simulink model "LoFT_Example3"  (R2024b)
settings: Solver=ode4  StartTime=0.0  StopTime=300  FixedStep=simu.dt  RelTol=1e-3
undefined symbols (not defined in the file): body, circtime, Communication, D1, Delta, irkb, line, LoFT, p0, Pn, s, simu, trip_time, Turbwind, waves, wind
libraries: simulink x350, spsThreePhaseVIMeasurementLib x41, spsThreePhasePISectionLineLib x34, spsThreePhaseParallelRLCLoadLib x21, spsThreePhaseTransformerTwoWindingsLib x14, spsLoadFlowBusLib x10, spsThreePhaseDynamicLoadLib x9, spsSynchronousMachinepuStandardLib x7, spsExcitationSystemLib x7, spsSteamTurbineandGovernorLib x7, spsGenericPowerSystemStabilizerLib x7, spsMultiBandPowerSystemStabilizerLib x7
(part 10 of 49)

== system LoFT_Example3/FOWT System/Subsystem7/wave series 9 ==
  1-D Lookup Table : Lookup_n-D  NumberOfTableDimensions=1  BreakpointsForDimension1=LoFT.Hydro.waveforces.time + 10  Table=squeeze(LoFT.Hydro.waveforces.force(1,1,:))  InternalRulePriority=Speed  RndMeth=Simplest
  1-D Lookup Table1 : Lookup_n-D  NumberOfTableDimensions=1  BreakpointsForDimension1=LoFT.Hydro.waveforces.time + 10  Table=squeeze(LoFT.Hydro.waveforces.force(1,2,:))  InternalRulePriority=Speed  RndMeth=Simplest
  1-D Lookup Table2 : Lookup_n-D  NumberOfTableDimensions=1  BreakpointsForDimension1=LoFT.Hydro.waveforces.time + 10  Table=squeeze(LoFT.Hydro.waveforces.force(1,3,:))  InternalRulePriority=Speed  RndMeth=Simplest
  Clock1 : Clock
  Clock2 : Clock
  Clock3 : Clock
  Vector Concatenate1 : Concatenate  NumInputs=3
  Out1 : Outport
  wires:
  1-D Lookup Table2/1 -> Vector Concatenate1/3
  1-D Lookup Table1/1 -> Vector Concatenate1/2
  Clock1/1 -> 1-D Lookup Table/1
  Clock3/1 -> 1-D Lookup Table2/1
  1-D Lookup Table/1 -> Vector Concatenate1/1
  Clock2/1 -> 1-D Lookup Table1/1
  Vector Concatenate1/1 -> Out1/1

== system LoFT_Example3/FOWT System/Wind Conditions/wind series 1 ==
  Clock1 : Clock
  Lookup Table2 : Lookup_n-D  NumberOfTableDimensions=1  BreakpointsForDimension1=Turbwind.WF(1).Time  BreakpointsForDimension2=wind.yDiscr  BreakpointsForDimension3=wind.zDiscr  Table=Turbwind.WF(1).WindVelX  InternalRulePriority=Speed  RndMeth=Simplest
  Out1 : Outport
  wires:
  Lookup Table2/1 -> Out1/1
  Clock1/1 -> Lookup Table2/1

== system LoFT_Example3/FOWT System/Wind Conditions/wind series 10 ==
  Clock1 : Clock
  Lookup Table2 : Lookup_n-D  NumberOfTableDimensions=1  BreakpointsForDimension1=Turbwind.WF(1).Time  BreakpointsForDimension2=wind.yDiscr  BreakpointsForDimension3=wind.zDiscr  Table=Turbwind.WF(10).WindVelX  InternalRulePriority=Speed  RndMeth=Simplest
  Scope : Scope
  Out1 : Outport
  wires:
  Clock1/1 -> Lookup Table2/1
  Lookup Table2/1 -> Scope/1, Out1/1

== system LoFT_Example3/FOWT System/Wind Conditions/wind series 11 ==
  Clock1 : Clock
  Lookup Table2 : Lookup_n-D  NumberOfTableDimensions=1  BreakpointsForDimension1=Turbwind.WF(1).Time  BreakpointsForDimension2=wind.yDiscr  BreakpointsForDimension3=wind.zDiscr  Table=Turbwind.WF(11).WindVelX  InternalRulePriority=Speed  RndMeth=Simplest
  Out1 : Outport
  wires:
  Lookup Table2/1 -> Out1/1
  Clock1/1 -> Lookup Table2/1

== system LoFT_Example3/FOWT System/Wind Conditions/wind series 12 ==
  Clock1 : Clock
  Lookup Table2 : Lookup_n-D  NumberOfTableDimensions=1  BreakpointsForDimension1=Turbwind.WF(1).Time  BreakpointsForDimension2=wind.yDiscr  BreakpointsForDimension3=wind.zDiscr  Table=Turbwind.WF(12).WindVelX  InternalRulePriority=Speed  RndMeth=Simplest
  Out1 : Outport
  wires:
  Clock1/1 -> Lookup Table2/1
  Lookup Table2/1 -> Out1/1

== system LoFT_Example3/FOWT System/Wind Conditions/wind series 13 ==
  Clock1 : Clock
  Lookup Table2 : Lookup_n-D  NumberOfTableDimensions=1  BreakpointsForDimension1=Turbwind.WF(1).Time  BreakpointsForDimension2=wind.yDiscr  BreakpointsForDimension3=wind.zDiscr  Table=Turbwind.WF(13).WindVelX  InternalRulePriority=Speed  RndMeth=Simplest
  Out1 : Outport
  wires:
  Lookup Table2/1 -> Out1/1
  Clock1/1 -> Lookup Table2/1

== system LoFT_Example3/FOWT System/Wind Conditions/wind series 14 ==
  Clock1 : Clock
  Lookup Table2 : Lookup_n-D  NumberOfTableDimensions=1  BreakpointsForDimension1=Turbwind.WF(1).Time  BreakpointsForDimension2=wind.yDiscr  BreakpointsForDimension3=wind.zDiscr  Table=Turbwind.WF(14).WindVelX  InternalRulePriority=Speed  RndMeth=Simplest
  Out1 : Outport
  wires:
  Clock1/1 -> Lookup Table2/1
  Lookup Table2/1 -> Out1/1

== system LoFT_Example3/FOWT System/Wind Conditions/wind series 15 ==
  Clock1 : Clock
  Lookup Table2 : Lookup_n-D  NumberOfTableDimensions=1  BreakpointsForDimension1=Turbwind.WF(1).Time  BreakpointsForDimension2=wind.yDiscr  BreakpointsForDimension3=wind.zDiscr  Table=Turbwind.WF(15).WindVelX  InternalRulePriority=Speed  RndMeth=Simplest
  Out1 : Outport
  wires:
  Lookup Table2/1 -> Out1/1
  Clock1/1 -> Lookup Table2/1

== system LoFT_Example3/FOWT System/Wind Conditions/wind series 16 ==
  Clock1 : Clock
  Lookup Table2 : Lookup_n-D  NumberOfTableDimensions=1  BreakpointsForDimension1=Turbwind.WF(1).Time  BreakpointsForDimension2=wind.yDiscr  BreakpointsForDimension3=wind.zDiscr  Table=Turbwind.WF(16).WindVelX  InternalRulePriority=Speed  RndMeth=Simplest
  Out1 : Outport
  wires:
  Clock1/1 -> Lookup Table2/1
  Lookup Table2/1 -> Out1/1

== system LoFT_Example3/FOWT System/Wind Conditions/wind series 17 ==
  Clock1 : Clock
  Lookup Table2 : Lookup_n-D  NumberOfTableDimensions=1  BreakpointsForDimension1=Turbwind.WF(1).Time  BreakpointsForDimension2=wind.yDiscr  BreakpointsForDimension3=wind.zDiscr  Table=Turbwind.WF(17).WindVelX  InternalRulePriority=Speed  RndMeth=Simplest
  Out1 : Outport
  wires:
  Lookup Table2/1 -> Out1/1
  Clock1/1 -> Lookup Table2/1

== system LoFT_Example3/FOWT System/Wind Conditions/wind series 18 ==
  Clock1 : Clock
  Lookup Table2 : Lookup_n-D  NumberOfTableDimensions=1  BreakpointsForDimension1=Turbwind.WF(1).Time  BreakpointsForDimension2=wind.yDiscr  BreakpointsForDimension3=wind.zDiscr  Table=Turbwind.WF(18).WindVelX  InternalRulePriority=Speed  RndMeth=Simplest
  Out1 : Outport
  wires:
  Clock1/1 -> Lookup Table2/1
  Lookup Table2/1 -> Out1/1

== system LoFT_Example3/FOWT System/Wind Conditions/wind series 19 ==
  Clock1 : Clock
  Lookup Table2 : Lookup_n-D  NumberOfTableDimensions=1  BreakpointsForDimension1=Turbwind.WF(1).Time  BreakpointsForDimension2=wind.yDiscr  BreakpointsForDimension3=wind.zDiscr  Table=Turbwind.WF(19).WindVelX  InternalRulePriority=Speed  RndMeth=Simplest
  Out1 : Outport
  wires:
  Lookup Table2/1 -> Out1/1
  Clock1/1 -> Lookup Table2/1

== system LoFT_Example3/FOWT System/Wind Conditions/wind series 2 ==
  Clock1 : Clock
  Lookup Table2 : Lookup_n-D  NumberOfTableDimensions=1  BreakpointsForDimension1=Turbwind.WF(1).Time  BreakpointsForDimension2=wind.yDiscr  BreakpointsForDimension3=wind.zDiscr  Table=Turbwind.WF(2).WindVelX  InternalRulePriority=Speed  RndMeth=Simplest
  Out1 : Outport
  wires:
  Clock1/1 -> Lookup Table2/1
  Lookup Table2/1 -> Out1/1

== system LoFT_Example3/FOWT System/Wind Conditions/wind series 20 ==
  Clock1 : Clock
  Lookup Table2 : Lookup_n-D  NumberOfTableDimensions=1  BreakpointsForDimension1=Turbwind.WF(1).Time  BreakpointsForDimension2=wind.yDiscr  BreakpointsForDimension3=wind.zDiscr  Table=Turbwind.WF(20).WindVelX  InternalRulePriority=Speed  RndMeth=Simplest
  Scope : Scope
  Out1 : Outport
  wires:
  Lookup Table2/1 -> Out1/1, Scope/1
  Clock1/1 -> Lookup Table2/1

== system LoFT_Example3/FOWT System/Wind Conditions/wind series 21 ==
  Clock1 : Clock
  Lookup Table2 : Lookup_n-D  NumberOfTableDimensions=1  BreakpointsForDimension1=Turbwind.WF(1).Time  BreakpointsForDimension2=wind.yDiscr  BreakpointsForDimension3=wind.zDiscr  Table=Turbwind.WF(21).WindVelX  InternalRulePriority=Speed  RndMeth=Simplest
  Out1 : Outport
  wires:
  Lookup Table2/1 -> Out1/1
  Clock1/1 -> Lookup Table2/1

== system LoFT_Example3/FOWT System/Wind Conditions/wind series 22 ==
  Clock1 : Clock
  Lookup Table2 : Lookup_n-D  NumberOfTableDimensions=1  BreakpointsForDimension1=Turbwind.WF(1).Time  BreakpointsForDimension2=wind.yDiscr  BreakpointsForDimension3=wind.zDiscr  Table=Turbwind.WF(22).WindVelX  InternalRulePriority=Speed  RndMeth=Simplest
  Out1 : Outport
  wires:
  Clock1/1 -> Lookup Table2/1
  Lookup Table2/1 -> Out1/1

== system LoFT_Example3/FOWT System/Wind Conditions/wind series 23 ==
  Clock1 : Clock
  Lookup Table2 : Lookup_n-D  NumberOfTableDimensions=1  BreakpointsForDimension1=Turbwind.WF(1).Time  BreakpointsForDimension2=wind.yDiscr  BreakpointsForDimension3=wind.zDiscr  Table=Turbwind.WF(23).WindVelX  InternalRulePriority=Speed  RndMeth=Simplest
  Out1 : Outport
  wires:
  Lookup Table2/1 -> Out1/1
  Clock1/1 -> Lookup Table2/1

== system LoFT_Example3/FOWT System/Wind Conditions/wind series 24 ==
  Clock1 : Clock
  Lookup Table2 : Lookup_n-D  NumberOfTableDimensions=1  BreakpointsForDimension1=Turbwind.WF(1).Time  BreakpointsForDimension2=wind.yDiscr  BreakpointsForDimension3=wind.zDiscr  Table=Turbwind.WF(24).WindVelX  InternalRulePriority=Speed  RndMeth=Simplest
  Out1 : Outport
  wires:
  Clock1/1 -> Lookup Table2/1
  Lookup Table2/1 -> Out1/1

== system LoFT_Example3/FOWT System/Wind Conditions/wind series 25 ==
  Clock1 : Clock
  Lookup Table2 : Lookup_n-D  NumberOfTableDimensions=1  BreakpointsForDimension1=Turbwind.WF(1).Time  BreakpointsForDimension2=wind.yDiscr  BreakpointsForDimension3=wind.zDiscr  Table=Turbwind.WF(25).WindVelX  InternalRulePriority=Speed  RndMeth=Simplest
  Out1 : Outport
  wires:
  Lookup Table2/1 -> Out1/1
  Clock1/1 -> Lookup Table2/1

== system LoFT_Example3/FOWT System/Wind Conditions/wind series 26 ==
  Clock1 : Clock
  Lookup Table2 : Lookup_n-D  NumberOfTableDimensions=1  BreakpointsForDimension1=Turbwind.WF(1).Time  BreakpointsForDimension2=wind.yDiscr  BreakpointsForDimension3=wind.zDiscr  Table=Turbwind.WF(26).WindVelX  InternalRulePriority=Speed  RndMeth=Simplest
  Out1 : Outport
  wires:
  Clock1/1 -> Lookup Table2/1
  Lookup Table2/1 -> Out1/1

== system LoFT_Example3/FOWT System/Wind Conditions/wind series 27 ==
  Clock1 : Clock
  Lookup Table2 : Lookup_n-D  NumberOfTableDimensions=1  BreakpointsForDimension1=Turbwind.WF(1).Time  BreakpointsForDimension2=wind.yDiscr  BreakpointsForDimension3=wind.zDiscr  Table=Turbwind.WF(27).WindVelX  InternalRulePriority=Speed  RndMeth=Simplest
  Out1 : Outport
  wires:
  Lookup Table2/1 -> Out1/1
  Clock1/1 -> Lookup Table2/1

== system LoFT_Example3/FOWT System/Wind Conditions/wind series 28 ==
  Clock1 : Clock
  Lookup Table2 : Lookup_n-D  NumberOfTableDimensions=1  BreakpointsForDimension1=Turbwind.WF(1).Time  BreakpointsForDimension2=wind.yDiscr  BreakpointsForDimension3=wind.zDiscr  Table=Turbwind.WF(28).WindVelX  InternalRulePriority=Speed  RndMeth=Simplest
  Out1 : Outport
  wires:
  Clock1/1 -> Lookup Table2/1
  Lookup Table2/1 -> Out1/1

== system LoFT_Example3/FOWT System/Wind Conditions/wind series 29 ==
  Clock1 : Clock
  Lookup Table2 : Lookup_n-D  NumberOfTableDimensions=1  BreakpointsForDimension1=Turbwind.WF(1).Time  BreakpointsForDimension2=wind.yDiscr  BreakpointsForDimension3=wind.zDiscr  Table=Turbwind.WF(29).WindVelX  InternalRulePriority=Speed  RndMeth=Simplest
  Out1 : Outport
  wires:
  Lookup Table2/1 -> Out1/1
  Clock1/1 -> Lookup Table2/1

== system LoFT_Example3/FOWT System/Wind Conditions/wind series 3 ==
  Clock1 : Clock
  Lookup Table2 : Lookup_n-D  NumberOfTableDimensions=1  BreakpointsForDimension1=Turbwind.WF(1).Time  BreakpointsForDimension2=wind.yDiscr  BreakpointsForDimension3=wind.zDiscr  Table=Turbwind.WF(3).WindVelX  InternalRulePriority=Speed  RndMeth=Simplest
  Out1 : Outport
  wires:
  Lookup Table2/1 -> Out1/1
  Clock1/1 -> Lookup Table2/1

== system LoFT_Example3/FOWT System/Wind Conditions/wind series 30 ==
  Clock1 : Clock
  Lookup Table2 : Lookup_n-D  NumberOfTableDimensions=1  BreakpointsForDimension1=Turbwind.WF(1).Time  BreakpointsForDimension2=wind.yDiscr  BreakpointsForDimension3=wind.zDiscr  Table=Turbwind.WF(30).WindVelX  InternalRulePriority=Speed  RndMeth=Simplest
  Scope : Scope
  Out1 : Outport
  wires:
  Lookup Table2/1 -> Out1/1, Scope/1
  Clock1/1 -> Lookup Table2/1

== system LoFT_Example3/FOWT System/Wind Conditions/wind series 31 ==
  Clock1 : Clock
  Lookup Table2 : Lookup_n-D  NumberOfTableDimensions=1  BreakpointsForDimension1=Turbwind.WF(1).Time  BreakpointsForDimension2=wind.yDiscr  BreakpointsForDimension3=wind.zDiscr  Table=Turbwind.WF(31).WindVelX  InternalRulePriority=Speed  RndMeth=Simplest
  Out1 : Outport
  wires:
  Lookup Table2/1 -> Out1/1
  Clock1/1 -> Lookup Table2/1

== system LoFT_Example3/FOWT System/Wind Conditions/wind series 32 ==
  Clock1 : Clock
  Lookup Table2 : Lookup_n-D  NumberOfTableDimensions=1  BreakpointsForDimension1=Turbwind.WF(1).Time  BreakpointsForDimension2=wind.yDiscr  BreakpointsForDimension3=wind.zDiscr  Table=Turbwind.WF(32).WindVelX  InternalRulePriority=Speed  RndMeth=Simplest
  Out1 : Outport
  wires:
  Clock1/1 -> Lookup Table2/1
  Lookup Table2/1 -> Out1/1

== system LoFT_Example3/FOWT System/Wind Conditions/wind series 33 ==
  Clock1 : Clock
  Lookup Table2 : Lookup_n-D  NumberOfTableDimensions=1  BreakpointsForDimension1=Turbwind.WF(1).Time  BreakpointsForDimension2=wind.yDiscr  BreakpointsForDimension3=wind.zDiscr  Table=Turbwind.WF(33).WindVelX  InternalRulePriority=Speed  RndMeth=Simplest
  Out1 : Outport
  wires:
  Lookup Table2/1 -> Out1/1
  Clock1/1 -> Lookup Table2/1

== system LoFT_Example3/FOWT System/Wind Conditions/wind series 34 ==
  Clock1 : Clock
  Lookup Table2 : Lookup_n-D  NumberOfTableDimensions=1  BreakpointsForDimension1=Turbwind.WF(1).Time  BreakpointsForDimension2=wind.yDiscr  BreakpointsForDimension3=wind.zDiscr  Table=Turbwind.WF(34).WindVelX  InternalRulePriority=Speed  RndMeth=Simplest
  Out1 : Outport
  wires:
  Clock1/1 -> Lookup Table2/1
  Lookup Table2/1 -> Out1/1

== system LoFT_Example3/FOWT System/Wind Conditions/wind series 35 ==
  Clock1 : Clock
  Lookup Table2 : Lookup_n-D  NumberOfTableDimensions=1  BreakpointsForDimension1=Turbwind.WF(1).Time  BreakpointsForDimension2=wind.yDiscr  BreakpointsForDimension3=wind.zDiscr  Table=Turbwind.WF(35).WindVelX  InternalRulePriority=Speed  RndMeth=Simplest
  Out1 : Outport
  wires:
  Lookup Table2/1 -> Out1/1
  Clock1/1 -> Lookup Table2/1

== system LoFT_Example3/FOWT System/Wind Conditions/wind series 36 ==
  Clock1 : Clock
  Lookup Table2 : Lookup_n-D  NumberOfTableDimensions=1  BreakpointsForDimension1=Turbwind.WF(1).Time  BreakpointsForDimension2=wind.yDiscr  BreakpointsForDimension3=wind.zDiscr  Table=Turbwind.WF(36).WindVelX  InternalRulePriority=Speed  RndMeth=Simplest
  Out1 : Outport
  wires:
  Clock1/1 -> Lookup Table2/1
  Lookup Table2/1 -> Out1/1

== system LoFT_Example3/FOWT System/Wind Conditions/wind series 37 ==
  Clock1 : Clock
  Lookup Table2 : Lookup_n-D  NumberOfTableDimensions=1  BreakpointsForDimension1=Turbwind.WF(1).Time  BreakpointsForDimension2=wind.yDiscr  BreakpointsForDimension3=wind.zDiscr  Table=Turbwind.WF(37).WindVelX  InternalRulePriority=Speed  RndMeth=Simplest
  Out1 : Outport
  wires:
  Lookup Table2/1 -> Out1/1
  Clock1/1 -> Lookup Table2/1

== system LoFT_Example3/FOWT System/Wind Conditions/wind series 38 ==
  Clock1 : Clock
  Lookup Table2 : Lookup_n-D  NumberOfTableDimensions=1  BreakpointsForDimension1=Turbwind.WF(1).Time  BreakpointsForDimension2=wind.yDiscr  BreakpointsForDimension3=wind.zDiscr  Table=Turbwind.WF(38).WindVelX  InternalRulePriority=Speed  RndMeth=Simplest
  Out1 : Outport
  wires:
  Clock1/1 -> Lookup Table2/1
  Lookup Table2/1 -> Out1/1

== system LoFT_Example3/FOWT System/Wind Conditions/wind series 39 ==
  Clock1 : Clock
  Lookup Table2 : Lookup_n-D  NumberOfTableDimensions=1  BreakpointsForDimension1=Turbwind.WF(1).Time  BreakpointsForDimension2=wind.yDiscr  BreakpointsForDimension3=wind.zDiscr  Table=Turbwind.WF(39).WindVelX  InternalRulePriority=Speed  RndMeth=Simplest
  Out1 : Outport
  wires:
  Lookup Table2/1 -> Out1/1
  Clock1/1 -> Lookup Table2/1

== system LoFT_Example3/FOWT System/Wind Conditions/wind series 4 ==
  Clock1 : Clock
  Lookup Table2 : Lookup_n-D  NumberOfTableDimensions=1  BreakpointsForDimension1=Turbwind.WF(1).Time  BreakpointsForDimension2=wind.yDiscr  BreakpointsForDimension3=wind.zDiscr  Table=Turbwind.WF(4).WindVelX  InternalRulePriority=Speed  RndMeth=Simplest
  Out1 : Outport
  wires:
  Clock1/1 -> Lookup Table2/1
  Lookup Table2/1 -> Out1/1

== system LoFT_Example3/FOWT System/Wind Conditions/wind series 40 ==
  Clock1 : Clock
  Lookup Table2 : Lookup_n-D  NumberOfTableDimensions=1  BreakpointsForDimension1=Turbwind.WF(1).Time  BreakpointsForDimension2=wind.yDiscr  BreakpointsForDimension3=wind.zDiscr  Table=Turbwind.WF(40).WindVelX  InternalRulePriority=Speed  RndMeth=Simplest
  Scope : Scope
  Out1 : Outport
  wires:
  Lookup Table2/1 -> Out1/1, Scope/1
  Clock1/1 -> Lookup Table2/1

== system LoFT_Example3/FOWT System/Wind Conditions/wind series 41 ==
  Clock1 : Clock
  Lookup Table2 : Lookup_n-D  NumberOfTableDimensions=1  BreakpointsForDimension1=Turbwind.WF(1).Time  BreakpointsForDimension2=wind.yDiscr  BreakpointsForDimension3=wind.zDiscr  Table=Turbwind.WF(41).WindVelX  InternalRulePriority=Speed  RndMeth=Simplest
  Out1 : Outport
  wires:
  Lookup Table2/1 -> Out1/1
  Clock1/1 -> Lookup Table2/1

== system LoFT_Example3/FOWT System/Wind Conditions/wind series 42 ==
  Clock1 : Clock
  Lookup Table2 : Lookup_n-D  NumberOfTableDimensions=1  BreakpointsForDimension1=Turbwind.WF(1).Time  BreakpointsForDimension2=wind.yDiscr  BreakpointsForDimension3=wind.zDiscr  Table=Turbwind.WF(42).WindVelX  InternalRulePriority=Speed  RndMeth=Simplest
  Out1 : Outport
  wires:
  Clock1/1 -> Lookup Table2/1
  Lookup Table2/1 -> Out1/1

== system LoFT_Example3/FOWT System/Wind Conditions/wind series 43 ==
  Clock1 : Clock
  Lookup Table2 : Lookup_n-D  NumberOfTableDimensions=1  BreakpointsForDimension1=Turbwind.WF(1).Time  BreakpointsForDimension2=wind.yDiscr  BreakpointsForDimension3=wind.zDiscr  Table=Turbwind.WF(43).WindVelX  InternalRulePriority=Speed  RndMeth=Simplest
  Out1 : Outport
  wires:
  Lookup Table2/1 -> Out1/1
  Clock1/1 -> Lookup Table2/1

== system LoFT_Example3/FOWT System/Wind Conditions/wind series 44 ==
  Clock1 : Clock
  Lookup Table2 : Lookup_n-D  NumberOfTableDimensions=1  BreakpointsForDimension1=Turbwind.WF(1).Time  BreakpointsForDimension2=wind.yDiscr  BreakpointsForDimension3=wind.zDiscr  Table=Turbwind.WF(44).WindVelX  InternalRulePriority=Speed  RndMeth=Simplest
  Out1 : Outport
  wires:
  Clock1/1 -> Lookup Table2/1
  Lookup Table2/1 -> Out1/1

== system LoFT_Example3/FOWT System/Wind Conditions/wind series 45 ==
  Clock1 : Clock
  Lookup Table2 : Lookup_n-D  NumberOfTableDimensions=1  BreakpointsForDimension1=Turbwind.WF(1).Time  BreakpointsForDimension2=wind.yDiscr  BreakpointsForDimension3=wind.zDiscr  Table=Turbwind.WF(45).WindVelX  InternalRulePriority=Speed  RndMeth=Simplest
  Out1 : Outport
  wires:
  Lookup Table2/1 -> Out1/1
  Clock1/1 -> Lookup Table2/1

== system LoFT_Example3/FOWT System/Wind Conditions/wind series 46 ==
  Clock1 : Clock
  Lookup Table2 : Lookup_n-D  NumberOfTableDimensions=1  BreakpointsForDimension1=Turbwind.WF(1).Time  BreakpointsForDimension2=wind.yDiscr  BreakpointsForDimension3=wind.zDiscr  Table=Turbwind.WF(46).WindVelX  InternalRulePriority=Speed  RndMeth=Simplest
  Out1 : Outport
  wires:
  Clock1/1 -> Lookup Table2/1
  Lookup Table2/1 -> Out1/1

== system LoFT_Example3/FOWT System/Wind Conditions/wind series 47 ==
  Clock1 : Clock
  Lookup Table2 : Lookup_n-D  NumberOfTableDimensions=1  BreakpointsForDimension1=Turbwind.WF(1).Time  BreakpointsForDimension2=wind.yDiscr  BreakpointsForDimension3=wind.zDiscr  Table=Turbwind.WF(47).WindVelX  InternalRulePriority=Speed  RndMeth=Simplest
  Out1 : Outport
  wires:
  Lookup Table2/1 -> Out1/1
  Clock1/1 -> Lookup Table2/1

== system LoFT_Example3/FOWT System/Wind Conditions/wind series 48 ==
  Clock1 : Clock
  Lookup Table2 : Lookup_n-D  NumberOfTableDimensions=1  BreakpointsForDimension1=Turbwind.WF(1).Time  BreakpointsForDimension2=wind.yDiscr  BreakpointsForDimension3=wind.zDiscr  Table=Turbwind.WF(48).WindVelX  InternalRulePriority=Speed  RndMeth=Simplest
  Out1 : Outport
  wires:
  Clock1/1 -> Lookup Table2/1
  Lookup Table2/1 -> Out1/1

== system LoFT_Example3/FOWT System/Wind Conditions/wind series 49 ==
  Clock1 : Clock
  Lookup Table2 : Lookup_n-D  NumberOfTableDimensions=1  BreakpointsForDimension1=Turbwind.WF(1).Time  BreakpointsForDimension2=wind.yDiscr  BreakpointsForDimension3=wind.zDiscr  Table=Turbwind.WF(49).WindVelX  InternalRulePriority=Speed  RndMeth=Simplest
  Out1 : Outport
  wires:
  Lookup Table2/1 -> Out1/1
  Clock1/1 -> Lookup Table2/1

== system LoFT_Example3/FOWT System/Wind Conditions/wind series 5 ==
  Clock1 : Clock
  Lookup Table2 : Lookup_n-D  NumberOfTableDimensions=1  BreakpointsForDimension1=Turbwind.WF(1).Time  BreakpointsForDimension2=wind.yDiscr  BreakpointsForDimension3=wind.zDiscr  Table=Turbwind.WF(5).WindVelX  InternalRulePriority=Speed  RndMeth=Simplest
  Out1 : Outport
  wires:
  Lookup Table2/1 -> Out1/1
  Clock1/1 -> Lookup Table2/1

== system LoFT_Example3/FOWT System/Wind Conditions/wind series 50 ==
  Clock1 : Clock
  Lookup Table2 : Lookup_n-D  NumberOfTableDimensions=1  BreakpointsForDimension1=Turbwind.WF(1).Time  BreakpointsForDimension2=wind.yDiscr  BreakpointsForDimension3=wind.zDiscr  Table=Turbwind.WF(50).WindVelX  InternalRulePriority=Speed  RndMeth=Simplest
  Scope : Scope
  Out1 : Outport
  wires:
  Lookup Table2/1 -> Out1/1, Scope/1
  Clock1/1 -> Lookup Table2/1

== system LoFT_Example3/FOWT System/Wind Conditions/wind series 51 ==
  Clock1 : Clock
  Lookup Table2 : Lookup_n-D  NumberOfTableDimensions=1  BreakpointsForDimension1=Turbwind.WF(1).Time  BreakpointsForDimension2=wind.yDiscr  BreakpointsForDimension3=wind.zDiscr  Table=Turbwind.WF(51).WindVelX  InternalRulePriority=Speed  RndMeth=Simplest
  Out1 : Outport
  wires:
  Lookup Table2/1 -> Out1/1
  Clock1/1 -> Lookup Table2/1

== system LoFT_Example3/FOWT System/Wind Conditions/wind series 52 ==
  Clock1 : Clock
  Lookup Table2 : Lookup_n-D  NumberOfTableDimensions=1  BreakpointsForDimension1=Turbwind.WF(1).Time  BreakpointsForDimension2=wind.yDiscr  BreakpointsForDimension3=wind.zDiscr  Table=Turbwind.WF(52).WindVelX  InternalRulePriority=Speed  RndMeth=Simplest
  Out1 : Outport
  wires:
  Clock1/1 -> Lookup Table2/1
  Lookup Table2/1 -> Out1/1

== system LoFT_Example3/FOWT System/Wind Conditions/wind series 53 ==
  Clock1 : Clock
  Lookup Table2 : Lookup_n-D  NumberOfTableDimensions=1  BreakpointsForDimension1=Turbwind.WF(1).Time  BreakpointsForDimension2=wind.yDiscr  BreakpointsForDimension3=wind.zDiscr  Table=Turbwind.WF(53).WindVelX  InternalRulePriority=Speed  RndMeth=Simplest
  Out1 : Outport
  wires:
  Lookup Table2/1 -> Out1/1
  Clock1/1 -> Lookup Table2/1

== system LoFT_Example3/FOWT System/Wind Conditions/wind series 54 ==
  Clock1 : Clock
  Lookup Table2 : Lookup_n-D  NumberOfTableDimensions=1  BreakpointsForDimension1=Turbwind.WF(1).Time  BreakpointsForDimension2=wind.yDiscr  BreakpointsForDimension3=wind.zDiscr  Table=Turbwind.WF(54).WindVelX  InternalRulePriority=Speed  RndMeth=Simplest
  Out1 : Outport
  wires:
  Clock1/1 -> Lookup Table2/1
  Lookup Table2/1 -> Out1/1

== system LoFT_Example3/FOWT System/Wind Conditions/wind series 55 ==
  Clock1 : Clock
  Lookup Table2 : Lookup_n-D  NumberOfTableDimensions=1  BreakpointsForDimension1=Turbwind.WF(1).Time  BreakpointsForDimension2=wind.yDiscr  BreakpointsForDimension3=wind.zDiscr  Table=Turbwind.WF(55).WindVelX  InternalRulePriority=Speed  RndMeth=Simplest
  Out1 : Outport
  wires:
  Lookup Table2/1 -> Out1/1
  Clock1/1 -> Lookup Table2/1

== system LoFT_Example3/FOWT System/Wind Conditions/wind series 56 ==
  Clock1 : Clock
  Lookup Table2 : Lookup_n-D  NumberOfTableDimensions=1  BreakpointsForDimension1=Turbwind.WF(1).Time  BreakpointsForDimension2=wind.yDiscr  BreakpointsForDimension3=wind.zDiscr  Table=Turbwind.WF(56).WindVelX  InternalRulePriority=Speed  RndMeth=Simplest
  Out1 : Outport
  wires:
  Clock1/1 -> Lookup Table2/1
  Lookup Table2/1 -> Out1/1

== system LoFT_Example3/FOWT System/Wind Conditions/wind series 57 ==
  Clock1 : Clock
  Lookup Table2 : Lookup_n-D  NumberOfTableDimensions=1  BreakpointsForDimension1=Turbwind.WF(1).Time  BreakpointsForDimension2=wind.yDiscr  BreakpointsForDimension3=wind.zDiscr  Table=Turbwind.WF(57).WindVelX  InternalRulePriority=Speed  RndMeth=Simplest
  Out1 : Outport
  wires:
  Lookup Table2/1 -> Out1/1
  Clock1/1 -> Lookup Table2/1

== system LoFT_Example3/FOWT System/Wind Conditions/wind series 58 ==
  Clock1 : Clock
  Lookup Table2 : Lookup_n-D  NumberOfTableDimensions=1  BreakpointsForDimension1=Turbwind.WF(1).Time  BreakpointsForDimension2=wind.yDiscr  BreakpointsForDimension3=wind.zDiscr  Table=Turbwind.WF(58).WindVelX  InternalRulePriority=Speed  RndMeth=Simplest
  Out1 : Outport
  wires:
  Clock1/1 -> Lookup Table2/1
  Lookup Table2/1 -> Out1/1

== system LoFT_Example3/FOWT System/Wind Conditions/wind series 59 ==
  Clock1 : Clock
  Lookup Table2 : Lookup_n-D  NumberOfTableDimensions=1  BreakpointsForDimension1=Turbwind.WF(1).Time  BreakpointsForDimension2=wind.yDiscr  BreakpointsForDimension3=wind.zDiscr  Table=Turbwind.WF(59).WindVelX  InternalRulePriority=Speed  RndMeth=Simplest
  Out1 : Outport
  wires:
  Lookup Table2/1 -> Out1/1
  Clock1/1 -> Lookup Table2/1

== system LoFT_Example3/FOWT System/Wind Conditions/wind series 6 ==
  Clock1 : Clock
  Lookup Table2 : Lookup_n-D  NumberOfTableDimensions=1  BreakpointsForDimension1=Turbwind.WF(1).Time  BreakpointsForDimension2=wind.yDiscr  BreakpointsForDimension3=wind.zDiscr  Table=Turbwind.WF(6).WindVelX  InternalRulePriority=Speed  RndMeth=Simplest
  Out1 : Outport
  wires:
  Clock1/1 -> Lookup Table2/1
  Lookup Table2/1 -> Out1/1

== system LoFT_Example3/FOWT System/Wind Conditions/wind series 60 ==
  Clock1 : Clock
  Lookup Table2 : Lookup_n-D  NumberOfTableDimensions=1  BreakpointsForDimension1=Turbwind.WF(1).Time  BreakpointsForDimension2=wind.yDiscr  BreakpointsForDimension3=wind.zDiscr  Table=Turbwind.WF(60).WindVelX  InternalRulePriority=Speed  RndMeth=Simplest
  Scope : Scope
  Out1 : Outport
  wires:
  Lookup Table2/1 -> Out1/1, Scope/1
  Clock1/1 -> Lookup Table2/1

== system LoFT_Example3/FOWT System/Wind Conditions/wind series 61 ==
  Clock1 : Clock
  Lookup Table2 : Lookup_n-D  NumberOfTableDimensions=1  BreakpointsForDimension1=Turbwind.WF(1).Time  BreakpointsForDimension2=wind.yDiscr  BreakpointsForDimension3=wind.zDiscr  Table=Turbwind.WF(61).WindVelX  InternalRulePriority=Speed  RndMeth=Simplest
  Out1 : Outport
  wires:
  Lookup Table2/1 -> Out1/1
  Clock1/1 -> Lookup Table2/1

== system LoFT_Example3/FOWT System/Wind Conditions/wind series 62 ==
  Clock1 : Clock
  Lookup Table2 : Lookup_n-D  NumberOfTableDimensions=1  BreakpointsForDimension1=Turbwind.WF(1).Time  BreakpointsForDimension2=wind.yDiscr  BreakpointsForDimension3=wind.zDiscr  Table=Turbwind.WF(62).WindVelX  InternalRulePriority=Speed  RndMeth=Simplest
  Out1 : Outport
  wires:
  Clock1/1 -> Lookup Table2/1
  Lookup Table2/1 -> Out1/1

== system LoFT_Example3/FOWT System/Wind Conditions/wind series 63 ==
  Clock1 : Clock
  Lookup Table2 : Lookup_n-D  NumberOfTableDimensions=1  BreakpointsForDimension1=Turbwind.WF(1).Time  BreakpointsForDimension2=wind.yDiscr  BreakpointsForDimension3=wind.zDiscr  Table=Turbwind.WF(63).WindVelX  InternalRulePriority=Speed  RndMeth=Simplest
  Out1 : Outport
  wires:
  Lookup Table2/1 -> Out1/1
  Clock1/1 -> Lookup Table2/1

== system LoFT_Example3/FOWT System/Wind Conditions/wind series 64 ==
  Clock1 : Clock
  Lookup Table2 : Lookup_n-D  NumberOfTableDimensions=1  BreakpointsForDimension1=Turbwind.WF(1).Time  BreakpointsForDimension2=wind.yDiscr  BreakpointsForDimension3=wind.zDiscr  Table=Turbwind.WF(64).WindVelX  InternalRulePriority=Speed  RndMeth=Simplest
  Out1 : Outport
  wires:
  Clock1/1 -> Lookup Table2/1
  Lookup Table2/1 -> Out1/1

== system LoFT_Example3/FOWT System/Wind Conditions/wind series 65 ==
  Clock1 : Clock
  Lookup Table2 : Lookup_n-D  NumberOfTableDimensions=1  BreakpointsForDimension1=Turbwind.WF(1).Time  BreakpointsForDimension2=wind.yDiscr  BreakpointsForDimension3=wind.zDiscr  Table=Turbwind.WF(65).WindVelX  InternalRulePriority=Speed  RndMeth=Simplest
  Out1 : Outport
  wires:
  Lookup Table2/1 -> Out1/1
  Clock1/1 -> Lookup Table2/1

== system LoFT_Example3/FOWT System/Wind Conditions/wind series 66 ==
  Clock1 : Clock
  Lookup Table2 : Lookup_n-D  NumberOfTableDimensions=1  BreakpointsForDimension1=Turbwind.WF(1).Time  BreakpointsForDimension2=wind.yDiscr  BreakpointsForDimension3=wind.zDiscr  Table=Turbwind.WF(66).WindVelX  InternalRulePriority=Speed  RndMeth=Simplest
  Out1 : Outport
  wires:
  Clock1/1 -> Lookup Table2/1
  Lookup Table2/1 -> Out1/1

== system LoFT_Example3/FOWT System/Wind Conditions/wind series 67 ==
  Clock1 : Clock
  Lookup Table2 : Lookup_n-D  NumberOfTableDimensions=1  BreakpointsForDimension1=Turbwind.WF(1).Time  BreakpointsForDimension2=wind.yDiscr  BreakpointsForDimension3=wind.zDiscr  Table=Turbwind.WF(67).WindVelX  InternalRulePriority=Speed  RndMeth=Simplest
  Out1 : Outport
  wires:
  Lookup Table2/1 -> Out1/1
  Clock1/1 -> Lookup Table2/1

== system LoFT_Example3/FOWT System/Wind Conditions/wind series 68 ==
  Clock1 : Clock
  Lookup Table2 : Lookup_n-D  NumberOfTableDimensions=1  BreakpointsForDimension1=Turbwind.WF(1).Time  BreakpointsForDimension2=wind.yDiscr  BreakpointsForDimension3=wind.zDiscr  Table=Turbwind.WF(68).WindVelX  InternalRulePriority=Speed  RndMeth=Simplest
  Out1 : Outport
  wires:
  Clock1/1 -> Lookup Table2/1
  Lookup Table2/1 -> Out1/1

== system LoFT_Example3/FOWT System/Wind Conditions/wind series 69 ==
  Clock1 : Clock
  Lookup Table2 : Lookup_n-D  NumberOfTableDimensions=1  BreakpointsForDimension1=Turbwind.WF(1).Time  BreakpointsForDimension2=wind.yDiscr  BreakpointsForDimension3=wind.zDiscr  Table=Turbwind.WF(69).WindVelX  InternalRulePriority=Speed  RndMeth=Simplest
  Out1 : Outport
  wires:
  Lookup Table2/1 -> Out1/1
  Clock1/1 -> Lookup Table2/1

== system LoFT_Example3/FOWT System/Wind Conditions/wind series 7 ==
  Clock1 : Clock
  Lookup Table2 : Lookup_n-D  NumberOfTableDimensions=1  BreakpointsForDimension1=Turbwind.WF(1).Time  BreakpointsForDimension2=wind.yDiscr  BreakpointsForDimension3=wind.zDiscr  Table=Turbwind.WF(7).WindVelX  InternalRulePriority=Speed  RndMeth=Simplest
  Out1 : Outport
  wires:
  Lookup Table2/1 -> Out1/1
  Clock1/1 -> Lookup Table2/1

== system LoFT_Example3/FOWT System/Wind Conditions/wind series 70 ==
  Clock1 : Clock
  Lookup Table2 : Lookup_n-D  NumberOfTableDimensions=1  BreakpointsForDimension1=Turbwind.WF(1).Time  BreakpointsForDimension2=wind.yDiscr  BreakpointsForDimension3=wind.zDiscr  Table=Turbwind.WF(70).WindVelX  InternalRulePriority=Speed  RndMeth=Simplest
  Scope : Scope
  Out1 : Outport
  wires:
  Lookup Table2/1 -> Out1/1, Scope/1
  Clock1/1 -> Lookup Table2/1

== system LoFT_Example3/FOWT System/Wind Conditions/wind series 8 ==
  Clock1 : Clock
  Lookup Table2 : Lookup_n-D  NumberOfTableDimensions=1  BreakpointsForDimension1=Turbwind.WF(1).Time  BreakpointsForDimension2=wind.yDiscr  BreakpointsForDimension3=wind.zDiscr  Table=Turbwind.WF(8).WindVelX  InternalRulePriority=Speed  RndMeth=Simplest
  Out1 : Outport
  wires:
  Clock1/1 -> Lookup Table2/1
  Lookup Table2/1 -> Out1/1

== system LoFT_Example3/FOWT System/Wind Conditions/wind series 9 ==
  Clock1 : Clock
  Lookup Table2 : Lookup_n-D  NumberOfTableDimensions=1  BreakpointsForDimension1=Turbwind.WF(1).Time  BreakpointsForDimension2=wind.yDiscr  BreakpointsForDimension3=wind.zDiscr  Table=Turbwind.WF(9).WindVelX  InternalRulePriority=Speed  RndMeth=Simplest
  Out1 : Outport
  wires:
  Lookup Table2/1 -> Out1/1
  Clock1/1 -> Lookup Table2/1
